simulink model "Dynamic_5R_xd_from_outside"  (R2019a)
settings: Solver=ode3  StartTime=0.0  StopTime=120  FixedStep=0.1  RelTol=1e-3
model workspace (MATLAB code in the model file):
  | fix_step = Simulink.Signal;
  | fix_step.DataType = 'double';
  | fix_step.Dimensions = 1;
  | fix_step.Complexity = 'real';
  | fix_step.SamplingMode = 'Sample based';
  | fix_step.InitialValue = '0.1';
values from neighbouring files (symbols this model uses):
  Kp = 7*eye(2)    [initial_Settings.m]
  Kv = 7*eye(2)    [initial_Settings.m]
  s = 0.0005.*s    [initial_Settings.m]    (also in number2.mat = [129 303 129.214546173 303.585228585 129.437661808 304.16472)
  s1 = [v1;v2]    [initial_Settings.m]
  s2 = [a1;a2]    [initial_Settings.m]
libraries: simulink x1
(part 2 of 2)

== matlab function Dynamic_5R_xd_from_outside/Codes ==
  data: xd input; vd input; ad input; dq input; q input; Kv input; Kp input; x output; t input; xd output; e output; Torque output; wq output; detJ output
function [x,xd,e,Torque,wq,detJ]=  armrobot( xd,vd,ad,dq,q,Kv,Kp,t)



% a1=2.5;
% a2=2.5;
% a3=2.5;
% a4=2.5;
% a5=2.0;


a1=0.25;
a2=0.25;
a3=0.25;
a4=0.25;
a5=0.20;


q2=q(1,1);
q5=q(2,1);

% fprintf('\n  theta2 = %f [rad]  and theta5= %f [rad] \n ' , q2, q5)


A=2*a2*a3*cos(q2)-2*a3*(a5*cos(q5)+a1);
B=2*a2*a3*sin(q2)-2*a3*a5*sin(q5);
C=-1*(-2*a2*(a5*cos(q5)+a1)*cos(q2)+2*a1*a5*cos(q5)-2*a2*sin(q2)*a5*sin(q5)+a1*a1+a2*a2+a3*a3+a5*a5-a4*a4);

t1 = (B+sqrt(A*A+B*B-C*C))/(A+C);

 t2= (B-sqrt(A*A+B*B-C*C))/(A+C);



q3 = 2*atan(t1);
q3 = 2*atan(t2);
q4 = atan2((a2*sin(q2)+a3*sin(q3)-a5*sin(q5)) ,(a2*cos(q2)+a3*cos(q3)-a1-a5*cos(q5)));



wq=[q2;q3;q4;q5];


%%Velocity
w2=dq(1,1);
w5=dq(2,1);


w=inv([-a3*sin(q3) , a4*sin(q4) ; a3*cos(q3) , -a4*cos(q4)])*[a2*w2*sin(q2)-a5*w5*sin(q5) ; -a2*w2*cos(q2)+a5*w5*cos(q5)];

w3=w(1,1);
w4=w(2,1);



%%%%%%%%%%%%%%%%%%%%%%%%%%











%% Acceleration

% alpha2=ddq(1,1);
% alpha5=ddq(2,1);
% 
% t2 = sin(q2);
% t4 = w2 ^ 2;
% t6 = cos(q2);
% t8 = w(1,1) ^ 2;
% t10 = cos(q3);
% t12 = w(2,1) ^ 2;
% t14 = cos(q4);
% t17 = sin(q5);
% t19 = w5 ^ 2;
% t21 = cos(q5);
% A1 = a2 * alpha2 * t2 + a2 * t4 * t6 + a3 * t8 * t10 - a4 * t12 * t14 - a5 * alpha5 * t17 - a5 * t19 * t21;
% 
% 
% t2 = cos(q2);
% t4 = w2 ^ 2;
% t6 = sin(q2);
% t8 = w(1,1) ^ 2;
% t10 = sin(q3);
% t12 = w(2,1) ^ 2;
% t14 = sin(q4);
% t17 = cos(q5);
% t19 = w5 ^ 2;
% t21 = sin(q5);
% A2 = -a2 * alpha2 * t2 + a2 * t4 * t6 + a3 * t8 * t10 - a4 * t12 * t14 + a5 * alpha5 * t17 - a5 * t19 * t21;
% 
% 
% 
% % This gives us alpha3 and alpha4
% alpha= inv([-a3*sin(q3) , a4*sin(q4) ; a3*cos(q3) , -a4*cos(q4)])*[A1;A2]
% 
% 


%% Jacobian Matrices
%Link2
% --------------------------------------------------------------
Jplink2=[-a2*0.5*sin(q2),0;a2*cos(q2)*0.5 , 0 ; 0, 0]
Jolink2=[0,0;0,0;1,0];
% --------------------------------------------------------------

%Link3
% --------------------------------------------------------------


%%Derivative theta3 wrt theta2
t1 = a3 * a2;
t2 = cos(q2);
t3 = t2 * t1;
t4 = 0.2e1 * t3;
t5 = cos(q5);
t7 = t5 * a5 + a1;
t8 = t7 * a3;
t9 = t3 - t8;
t11 = sin(q2);
t12 = t11 * t1;
t13 = sin(q5);
t15 = a5 * a3 * t13;
t16 = t12 - t15;
t18 = t7 * a2;
t20 = 0.2e1 * t2 * t18;
t23 = 0.2e1 * a5 * a1 * t5;
t25 = a2 * a5;
t27 = 0.2e1 * t25 * t13 * t11;
t28 = a1 ^ 2;
t29 = a2 ^ 2;
t30 = a3 ^ 2;
t31 = a5 ^ 2;
t32 = a4 ^ 2;
t33 = t20 - t23 + t27 - t28 - t29 - t30 - t31 + t32;
t34 = t33 ^ 2;
t36 = sqrt(0.4e1 * t16 ^ 2 + 0.4e1 * t9 ^ 2 - t34);
t46 = t11 * t18;
t48 = t25 * t13 * t2;
t57 = t4 - 0.2e1 * t8 + t20 - t23 + t27 - t28 - t29 - t30 - t31 + t32;
t62 = 0.2e1 * t12 - 0.2e1 * t15 - t36;
t63 = t57 ^ 2;
t64 = 0.1e1 / t63;
t69 = t62 ^ 2;
derivative_q3_wrt_q2= 0.2e1 / (t64 * t69 + 0.1e1) * (0.1e1 / t57 * (t4 - (-0.8e1 * t11 * a3 * a2 * t9 + 0.8e1 * t2 * a3 * a2 * t16 - 0.4e1 * (-t46 + t48) * t33) / t36 / 0.2e1) - 0.2e1 * (-t12 - t46 + t48) * t64 * t62);



%%Derivative theta3 wrt theta5


t1 = cos(q5);
t5 = a3 * a2;
t6 = cos(q2);
t7 = t6 * t5;
t9 = t1 * a5 + a1;
t10 = t9 * a3;
t11 = t7 - t10;
t13 = sin(q2);
t14 = t13 * t5;
t15 = sin(q5);
t17 = a5 * a3 * t15;
t18 = t14 - t17;
t22 = 0.2e1 * t6 * t9 * a2;
t25 = 0.2e1 * a5 * a1 * t1;
t27 = a2 * a5;
t29 = 0.2e1 * t27 * t15 * t13;
t30 = a1 ^ 2;
t31 = a2 ^ 2;
t32 = a3 ^ 2;
t33 = a5 ^ 2;
t34 = a4 ^ 2;
t35 = t22 - t25 + t29 - t30 - t31 - t32 - t33 + t34;
t36 = t35 ^ 2;
t38 = sqrt(0.4e1 * t11 ^ 2 + 0.4e1 * t18 ^ 2 - t36);
t41 = a3 * a5;
t48 = t27 * t15 * t6;
t50 = a5 * a1 * t15;
t52 = t27 * t1 * t13;
t62 = 0.2e1 * t7 - 0.2e1 * t10 + t22 - t25 + t29 - t30 - t31 - t32 - t33 + t34;
t67 = 0.2e1 * t14 - 0.2e1 * t17 - t38;
t68 = t62 ^ 2;
t69 = 0.1e1 / t68;
t74 = t67 ^ 2;
derivative_q3_wrt_q5 = 0.2e1 / (t69 * t74 + 0.1e1) * (0.1e1 / t62 * (-0.2e1 * a5 * a3 * t1 - (0.8e1 * t41 * t15 * t11 - 0.8e1 * t41 * t1 * t18 - 0.4e1 * (-t48 + t50 + t52) * t35) / t38 / 0.2e1) - 0.2e1 * (t17 - t48 + t50 + t52) * t69 * t67);






Jplink3=[-a2*sin(q2)-a3*0.5*sin(q3)*derivative_q3_wrt_q2 , -a3*0.5*sin(q3)*derivative_q3_wrt_q5 ;
          a2*cos(q2)+a3*0.5*cos(q3)*derivative_q3_wrt_q2 , a3*0.5*cos(q3)*derivative_q3_wrt_q5;
           0     , 0];

Jolink3=[0,0;0,0;derivative_q3_wrt_q2,derivative_q3_wrt_q5];
% --------------------------------------------------------------


% link4
% --------------------------------------------------------------
%%Derivative theta4 wrt theta2
t1 = cos(q2);
t2 = a2 * t1;
t3 = a3 * a2;
t4 = t1 * t3;
t5 = 0.2e1 * t4;
t6 = cos(q5);
t7 = t6 * a5;
t8 = t7 + a1;
t9 = t8 * a3;
t10 = t4 - t9;
t12 = sin(q2);
t13 = t12 * t3;
t14 = sin(q5);
t16 = a5 * a3 * t14;
t17 = t13 - t16;
t19 = t8 * a2;
t21 = 0.2e1 * t1 * t19;
t24 = 0.2e1 * a5 * a1 * t6;
t26 = a2 * a5;
t28 = 0.2e1 * t26 * t14 * t12;
t29 = a1 ^ 2;
t30 = a2 ^ 2;
t31 = a3 ^ 2;
t32 = a5 ^ 2;
t33 = a4 ^ 2;
t34 = t21 - t24 + t28 - t29 - t30 - t31 - t32 + t33;
t35 = t34 ^ 2;
t37 = sqrt(0.4e1 * t10 ^ 2 + 0.4e1 * t17 ^ 2 - t35);
t47 = t12 * t19;
t49 = t26 * t14 * t1;
t58 = t5 - 0.2e1 * t9 + t21 - t24 + t28 - t29 - t30 - t31 - t32 + t33;
t59 = 0.1e1 / t58;
t63 = 0.2e1 * t13 - 0.2e1 * t16 - t37;
t64 = t58 ^ 2;
t65 = 0.1e1 / t64;
t70 = (t59 * (t5 - (-0.8e1 * t12 * a3 * a2 * t10 + 0.8e1 * t1 * a3 * a2 * t17 - 0.4e1 * (-t47 + t49) * t34) / t37 / 0.2e1) - 0.2e1 * (-t13 - t47 + t49) * t65 * t63) * a3;
t71 = t63 ^ 2;
t74 = 0.1e1 / (t65 * t71 + 0.1e1);
t76 = atan(t59 * t63);
t77 = 0.2e1 * t76;
t78 = cos(t77);
t84 = t78 * a3 - a1 + t2 - t7;
t87 = t12 * a2;
t88 = sin(t77);
t91 = t88 * a3 - t14 * a5 + t87;
t92 = t91 ^ 2;
t93 = t84 ^ 2;
t94 = 0.1e1 / t93;
t97 = 0.1e1 / (t94 * t92 + 0.1e1);
derivative_q4_wrt_q2 = t97 / t84 * (0.2e1 * t78 * t74 * t70 + t2) - t97 * t94 * t91 * (-0.2e1 * t88 * t74 * t70 - t87);





%%Derivative theta4 wrt theta5


t1 = cos(q5);
t5 = a3 * a2;
t6 = cos(q2);
t7 = t6 * t5;
t8 = t1 * a5;
t9 = t8 + a1;
t10 = t9 * a3;
t11 = t7 - t10;
t13 = sin(q2);
t14 = t13 * t5;
t15 = sin(q5);
t17 = a5 * a3 * t15;
t18 = t14 - t17;
t22 = 0.2e1 * t6 * t9 * a2;
t25 = 0.2e1 * a5 * a1 * t1;
t27 = a2 * a5;
t29 = 0.2e1 * t27 * t15 * t13;
t30 = a1 ^ 2;
t31 = a2 ^ 2;
t32 = a3 ^ 2;
t33 = a5 ^ 2;
t34 = a4 ^ 2;
t35 = t22 - t25 + t29 - t30 - t31 - t32 - t33 + t34;
t36 = t35 ^ 2;
t38 = sqrt(0.4e1 * t11 ^ 2 + 0.4e1 * t18 ^ 2 - t36);
t41 = a3 * a5;
t48 = t27 * t15 * t6;
t50 = a5 * a1 * t15;
t52 = t27 * t1 * t13;
t62 = 0.2e1 * t7 - 0.2e1 * t10 + t22 - t25 + t29 - t30 - t31 - t32 - t33 + t34;
t63 = 0.1e1 / t62;
t67 = 0.2e1 * t14 - 0.2e1 * t17 - t38;
t68 = t62 ^ 2;
t69 = 0.1e1 / t68;
t74 = ((-0.2e1 * a5 * a3 * t1 - (0.8e1 * t41 * t15 * t11 - 0.8e1 * t41 * t1 * t18 - 0.4e1 * (-t48 + t50 + t52) * t35) / t38 / 0.2e1) * t63 - 0.2e1 * (t17 - t48 + t50 + t52) * t69 * t67) * a3;
t75 = t67 ^ 2;
t78 = 0.1e1 / (t69 * t75 + 0.1e1);
t80 = atan(t63 * t67);
t81 = 0.2e1 * t80;
t82 = cos(t81);
t89 = a2 * t6 + t82 * a3 - a1 - t8;
t93 = sin(t81);
t95 = t15 * a5;
t96 = t13 * a2 + t93 * a3 - t95;
t97 = t96 ^ 2;
t98 = t89 ^ 2;
t99 = 0.1e1 / t98;
t102 = 0.1e1 / (t99 * t97 + 0.1e1);
derivative_q4_wrt_q5= 0.1e1 / t89 * (0.2e1 * t82 * t78 * t74 - t8) * t102 - t102 * t99 * t96 * (-0.2e1 * t93 * t78 * t74 + t95);

Jplink4=[-a4*0.5*sin(q4)*derivative_q4_wrt_q2 , -a5*sin(q5)-a4*0.5*sin(q4)*derivative_q4_wrt_q5 ;
         a4*0.5*cos(q4)*derivative_q4_wrt_q2 , a5*cos(q5)+a4*0.5*cos(q4)*derivative_q4_wrt_q5 ; 0,0];


     
Jolink4=[0,0 ; 0,0 ; derivative_q4_wrt_q2 ,derivative_q4_wrt_q5];     
     
% link5   
Jplink5=[0,-a5*0.5*sin(q5) ; 0 ,a5*0.5*cos(q5) ; 0 ,0];
Jolink5=[0,0;0,0;0,1];










%%Second Derivatives


% Derivative of function q3 with respect to q2 q2


t1 = a2 * a3;
t2 = sin(q2);
t3 = t2 * t1;
t4 = 0.2e1 * t3;
t5 = cos(q2);
t6 = t5 * t1;
t7 = cos(q5);
t9 = t7 * a5 + a1;
t10 = t9 * a3;
t11 = t6 - t10;
t12 = 0.2e1 * a2 * t11;
t13 = t2 * a3;
t16 = sin(q5);
t18 = a5 * a3 * t16;
t19 = t3 - t18;
t20 = 0.2e1 * a2 * t19;
t21 = t5 * a3;
t24 = t9 * a2;
t25 = t5 * t24;
t26 = 0.2e1 * t25;
t29 = 0.2e1 * a5 * a1 * t7;
t31 = a2 * a5;
t32 = t31 * t16 * t2;
t33 = 0.2e1 * t32;
t34 = a1 ^ 2;
t35 = a2 ^ 2;
t36 = a3 ^ 2;
t37 = a5 ^ 2;
t38 = a4 ^ 2;
t39 = t26 - t29 + t33 - t34 - t35 - t36 - t37 + t38;
t40 = t2 * t24;
t42 = t31 * t16 * t5;
t43 = -t40 + t42;
t46 = -0.4e1 * t13 * t12 + 0.4e1 * t21 * t20 - 0.4e1 * t43 * t39;
t47 = t46 ^ 2;
t50 = t39 ^ 2;
t51 = 0.4e1 * t11 ^ 2 + 0.4e1 * t19 ^ 2 - t50;
t52 = sqrt(t51);
t57 = t2 ^ 2;
t63 = t5 ^ 2;
t75 = 0.1e1 / t52;
t79 = 0.2e1 * t6;
t81 = t79 - 0.2e1 * t10 + t26 - t29 + t33 - t34 - t35 - t36 - t37 + t38;
t82 = 0.1e1 / t81;
t86 = t79 - t75 * t46 / 0.2e1;
t87 = -t3 - t40 + t42;
t89 = t81 ^ 2;
t90 = 0.1e1 / t89;
t94 = t4 - 0.2e1 * t18 - t52;
t98 = 0.1e1 / t89 / t81;
t105 = t94 ^ 2;
t107 = t90 * t105 + 0.1e1;
t120 = t107 ^ 2;
derivative_q3_wrt_q2_q2 = 0.2e1 / t107 * (t82 * (-t4 + 0.1e1 / t52 / t51 * t47 / 0.4e1 - t75 * (0.8e1 * t36 * t35 * t57 - 0.4e1 * t21 * t12 + 0.8e1 * t36 * t35 * t63 - 0.4e1 * t13 * t20 - 0.8e1 * t43 ^ 2 - 0.4e1 * (-t25 - t32) * t39) / 0.2e1) - 0.4e1 * t90 * t87 * t86 + 0.8e1 * t98 * t87 ^ 2 * t94 - 0.2e1 * t90 * (-t6 - t25 - t32) * t94) - 0.4e1 / t120 * (-0.2e1 * t98 * t87 * t105 + t90 * t86 * t94) * (-0.2e1 * t90 * t87 * t94 + t82 * t86);





% derivative q3 with respecto q2 q5



t1 = a3 * a2;
t2 = cos(q2);
t3 = t2 * t1;
t4 = cos(q5);
t6 = t4 * a5 + a1;
t7 = t6 * a3;
t8 = t3 - t7;
t10 = sin(q2);
t14 = t10 * t1;
t15 = sin(q5);
t17 = a5 * a3 * t15;
t18 = t14 - t17;
t23 = t6 * a2;
t25 = 0.2e1 * t2 * t23;
t28 = 0.2e1 * a5 * a1 * t4;
t29 = t15 * t10;
t30 = a2 * a5;
t31 = t30 * t29;
t32 = 0.2e1 * t31;
t33 = a1 ^ 2;
t34 = a2 ^ 2;
t35 = a3 ^ 2;
t36 = a5 ^ 2;
t37 = a4 ^ 2;
t38 = t25 - t28 + t32 - t33 - t34 - t35 - t36 + t37;
t39 = t10 * t23;
t41 = t30 * t15 * t2;
t42 = -t39 + t41;
t45 = -0.8e1 * t10 * a3 * a2 * t8 + 0.8e1 * t2 * a3 * a2 * t18 - 0.4e1 * t42 * t38;
t47 = a3 * a5;
t54 = a5 * a1 * t15;
t56 = t30 * t4 * t10;
t57 = -t41 + t54 + t56;
t60 = 0.8e1 * t47 * t15 * t8 - 0.8e1 * t47 * t4 * t18 - 0.4e1 * t57 * t38;
t64 = t38 ^ 2;
t65 = 0.4e1 * t18 ^ 2 + 0.4e1 * t8 ^ 2 - t64;
t66 = sqrt(t65);
t72 = a5 * t35 * a2;
t75 = t4 * t2;
t81 = t30 * t75 + t31;
t85 = 0.1e1 / t66;
t89 = 0.2e1 * t3;
t91 = t89 - 0.2e1 * t7 + t25 - t28 + t32 - t33 - t34 - t35 - t36 + t37;
t92 = 0.1e1 / t91;
t96 = t89 - t85 * t45 / 0.2e1;
t97 = t17 - t41 + t54 + t56;
t99 = t91 ^ 2;
t100 = 0.1e1 / t99;
t107 = -0.2e1 * a5 * a3 * t4 - t85 * t60 / 0.2e1;
t108 = -t14 - t39 + t41;
t113 = 0.2e1 * t14 - 0.2e1 * t17 - t66;
t114 = 0.2e1 * t108 * t113;
t116 = 0.1e1 / t99 / t91;
t123 = t113 ^ 2;
t125 = t100 * t123 + 0.1e1;
t137 = t125 ^ 2;
derivative_q3_wrt_q2_q5 = 0.2e1 / t125 * (t92 * (0.1e1 / t66 / t65 * t60 * t45 / 0.4e1 - t85 * (-0.8e1 * t72 * t29 - 0.4e1 * t81 * t38 - 0.8e1 * t42 * t57 - 0.8e1 * t72 * t75) / 0.2e1) - 0.2e1 * t100 * t97 * t96 - 0.2e1 * t100 * t108 * t107 + 0.4e1 * t116 * t97 * t114 - 0.2e1 * t100 * t81 * t113) - 0.4e1 / t137 * (t100 * t107 * t113 - 0.2e1 * t116 * t97 * t123) * (-t100 * t114 + t92 * t96);


%derivative q3 with respecto q5 q5

t1 = sin(q5);
t3 = a5 * a3 * t1;
t4 = 0.2e1 * t3;
t5 = a2 * a3;
t6 = cos(q2);
t7 = t6 * t5;
t8 = cos(q5);
t10 = t8 * a5 + a1;
t11 = t10 * a3;
t12 = t7 - t11;
t14 = a3 * a5;
t17 = sin(q2);
t18 = t17 * t5;
t19 = t18 - t3;
t25 = 0.2e1 * t6 * t10 * a2;
t27 = a5 * a1 * t8;
t28 = 0.2e1 * t27;
t30 = a2 * a5;
t31 = t30 * t1 * t17;
t32 = 0.2e1 * t31;
t33 = a1 ^ 2;
t34 = a2 ^ 2;
t35 = a3 ^ 2;
t36 = a5 ^ 2;
t37 = a4 ^ 2;
t38 = t25 - t28 + t32 - t33 - t34 - t35 - t36 + t37;
t40 = t30 * t1 * t6;
t42 = a5 * a1 * t1;
t44 = t30 * t8 * t17;
t45 = -t40 + t42 + t44;
t48 = 0.8e1 * t14 * t1 * t12 - 0.8e1 * t14 * t8 * t19 - 0.4e1 * t45 * t38;
t49 = t48 ^ 2;
t52 = t38 ^ 2;
t53 = 0.4e1 * t12 ^ 2 + 0.4e1 * t19 ^ 2 - t52;
t54 = sqrt(t53);
t59 = t1 ^ 2;
t66 = t8 ^ 2;
t76 = t30 * t8 * t6;
t81 = 0.1e1 / t54;
t87 = 0.2e1 * t7 - 0.2e1 * t11 + t25 - t28 + t32 - t33 - t34 - t35 - t36 + t37;
t88 = 0.1e1 / t87;
t91 = a5 * a3 * t8;
t95 = -0.2e1 * t91 - t81 * t48 / 0.2e1;
t96 = t3 - t40 + t42 + t44;
t98 = t87 ^ 2;
t99 = 0.1e1 / t98;
t103 = 0.2e1 * t18 - t4 - t54;
t107 = 0.1e1 / t98 / t87;
t114 = t103 ^ 2;
t116 = t99 * t114 + 0.1e1;
t129 = t116 ^ 2;
derivative_q3_wrt_q5_q5 = 0.2e1 / t116 * (t88 * (t4 + 0.1e1 / t54 / t53 * t49 / 0.4e1 - t81 * (0.8e1 * t36 * t35 * t59 + 0.8e1 * t14 * t8 * t12 + 0.8e1 * t36 * t35 * t66 + 0.8e1 * t14 * t1 * t19 - 0.8e1 * t45 ^ 2 - 0.4e1 * (-t76 + t27 - t31) * t38) / 0.2e1) - 0.4e1 * t99 * t96 * t95 + 0.8e1 * t107 * t96 ^ 2 * t103 - 0.2e1 * t99 * (t91 - t76 + t27 - t31) * t103) - 0.4e1 / t129 * (t99 * t95 * t103 - 0.2e1 * t107 * t96 * t114) * (-0.2e1 * t99 * t96 * t103 + t88 * t95);

%%%%



%-------------------------------------------------
% derivative theta4 with respect to theta2 theta2

t1 = sin(q2);
t2 = t1 * a2;
t3 = a3 * a2;
t4 = t1 * t3;
t5 = 0.2e1 * t4;
t6 = cos(q2);
t7 = t6 * t3;
t8 = cos(q5);
t9 = t8 * a5;
t10 = t9 + a1;
t11 = t10 * a3;
t12 = t7 - t11;
t13 = 0.2e1 * a2 * t12;
t14 = t1 * a3;
t17 = sin(q5);
t19 = a5 * a3 * t17;
t20 = t4 - t19;
t21 = 0.2e1 * a2 * t20;
t22 = t6 * a3;
t25 = t10 * a2;
t26 = t6 * t25;
t27 = 0.2e1 * t26;
t30 = 0.2e1 * a5 * a1 * t8;
t32 = a2 * a5;
t33 = t32 * t17 * t1;
t34 = 0.2e1 * t33;
t35 = a1 ^ 2;
t36 = a2 ^ 2;
t37 = a3 ^ 2;
t38 = a5 ^ 2;
t39 = a4 ^ 2;
t40 = t27 - t30 + t34 - t35 - t36 - t37 - t38 + t39;
t41 = t1 * t25;
t43 = t32 * t17 * t6;
t44 = -t41 + t43;
t47 = -0.4e1 * t14 * t13 + 0.4e1 * t22 * t21 - 0.4e1 * t44 * t40;
t48 = t47 ^ 2;
t51 = t40 ^ 2;
t52 = 0.4e1 * t12 ^ 2 + 0.4e1 * t20 ^ 2 - t51;
t53 = sqrt(t52);
t58 = t1 ^ 2;
t64 = t6 ^ 2;
t76 = 0.1e1 / t53;
t80 = 0.2e1 * t7;
t82 = t80 - 0.2e1 * t11 + t27 - t30 + t34 - t35 - t36 - t37 - t38 + t39;
t83 = 0.1e1 / t82;
t87 = t80 - t76 * t47 / 0.2e1;
t88 = -t4 - t41 + t43;
t90 = t82 ^ 2;
t91 = 0.1e1 / t90;
t95 = t5 - 0.2e1 * t19 - t53;
t99 = 0.1e1 / t90 / t82;
t106 = (t83 * (-t5 + 0.1e1 / t53 / t52 * t48 / 0.4e1 - t76 * (0.8e1 * t37 * t36 * t58 - 0.4e1 * t22 * t13 + 0.8e1 * t37 * t36 * t64 - 0.4e1 * t14 * t21 - 0.8e1 * t44 ^ 2 - 0.4e1 * (-t26 - t33) * t40) / 0.2e1) - 0.4e1 * t91 * t88 * t87 + 0.8e1 * t99 * t88 ^ 2 * t95 - 0.2e1 * t91 * (-t7 - t26 - t33) * t95) * a3;
t108 = atan(t83 * t95);
t109 = 0.2e1 * t108;
t110 = cos(t109);
t111 = t95 ^ 2;
t113 = t91 * t111 + 0.1e1;
t114 = 0.1e1 / t113;
t115 = t114 * t110;
t121 = -0.2e1 * t91 * t88 * t95 + t83 * t87;
t122 = t121 * a3;
t127 = -0.2e1 * t99 * t88 * t111 + t91 * t87 * t95;
t129 = t113 ^ 2;
t130 = 0.1e1 / t129;
t134 = t121 ^ 2;
t135 = t134 * a3;
t136 = sin(t109);
t141 = t6 * a2;
t143 = t110 * a3 - a1 + t141 - t9;
t144 = 0.1e1 / t143;
t148 = t136 * a3 - t17 * a5 + t2;
t149 = t148 ^ 2;
t150 = t143 ^ 2;
t151 = 0.1e1 / t150;
t153 = t151 * t149 + 0.1e1;
t154 = 0.1e1 / t153;
t158 = 0.2e1 * t115 * t122 + t141;
t159 = t114 * t136;
t162 = -0.2e1 * t159 * t122 - t2;
t164 = t154 * t151;
t171 = 0.1e1 / t150 / t143;
t173 = t151 * t158 * t148 - t171 * t162 * t149;
t175 = t153 ^ 2;
t176 = 0.1e1 / t175;
t191 = t162 ^ 2;
derivative_q4_wrt_q2_q2 = t154 * t144 * (-0.4e1 * t130 * t127 * t110 * t122 - 0.4e1 * t130 * t136 * t135 + 0.2e1 * t115 * t106 - t2) - 0.2e1 * t164 * t162 * t158 - 0.2e1 * t176 * t144 * t173 * t158 - t164 * t148 * (0.4e1 * t130 * t127 * t136 * t122 - 0.4e1 * t130 * t110 * t135 - 0.2e1 * t159 * t106 - t141) + 0.2e1 * t154 * t171 * t148 * t191 + 0.2e1 * t176 * t151 * t173 * t148 * t162;

%-------------------------------------------------------------
% derivative theta4 with respect to theta2 theta5




t1 = a3 * a2;
t2 = cos(q2);
t3 = t2 * t1;
t4 = cos(q5);
t5 = t4 * a5;
t6 = t5 + a1;
t7 = t6 * a3;
t8 = t3 - t7;
t10 = sin(q2);
t14 = t10 * t1;
t15 = sin(q5);
t17 = a5 * a3 * t15;
t18 = t14 - t17;
t23 = t6 * a2;
t25 = 0.2e1 * t2 * t23;
t28 = 0.2e1 * a5 * a1 * t4;
t29 = t15 * t10;
t30 = a2 * a5;
t31 = t30 * t29;
t32 = 0.2e1 * t31;
t33 = a1 ^ 2;
t34 = a2 ^ 2;
t35 = a3 ^ 2;
t36 = a5 ^ 2;
t37 = a4 ^ 2;
t38 = t25 - t28 + t32 - t33 - t34 - t35 - t36 + t37;
t39 = t10 * t23;
t41 = t30 * t15 * t2;
t42 = -t39 + t41;
t45 = -0.8e1 * t10 * a3 * a2 * t8 + 0.8e1 * t2 * a3 * a2 * t18 - 0.4e1 * t42 * t38;
t47 = a3 * a5;
t54 = a5 * a1 * t15;
t56 = t30 * t4 * t10;
t57 = -t41 + t54 + t56;
t60 = 0.8e1 * t47 * t15 * t8 - 0.8e1 * t47 * t4 * t18 - 0.4e1 * t57 * t38;
t64 = t38 ^ 2;
t65 = 0.4e1 * t18 ^ 2 + 0.4e1 * t8 ^ 2 - t64;
t66 = sqrt(t65);
t72 = a5 * t35 * a2;
t75 = t4 * t2;
t81 = t30 * t75 + t31;
t85 = 0.1e1 / t66;
t89 = 0.2e1 * t3;
t91 = t89 - 0.2e1 * t7 + t25 - t28 + t32 - t33 - t34 - t35 - t36 + t37;
t92 = 0.1e1 / t91;
t96 = t89 - t85 * t45 / 0.2e1;
t97 = t17 - t41 + t54 + t56;
t99 = t91 ^ 2;
t100 = 0.1e1 / t99;
t107 = -0.2e1 * a5 * a3 * t4 - t85 * t60 / 0.2e1;
t108 = -t14 - t39 + t41;
t113 = 0.2e1 * t14 - 0.2e1 * t17 - t66;
t114 = 0.2e1 * t108 * t113;
t116 = 0.1e1 / t99 / t91;
t123 = (t92 * (0.1e1 / t66 / t65 * t60 * t45 / 0.4e1 - t85 * (-0.8e1 * t72 * t29 - 0.4e1 * t81 * t38 - 0.8e1 * t42 * t57 - 0.8e1 * t72 * t75) / 0.2e1) - 0.2e1 * t100 * t97 * t96 - 0.2e1 * t100 * t108 * t107 + 0.4e1 * t116 * t97 * t114 - 0.2e1 * t100 * t81 * t113) * a3;
t125 = atan(t92 * t113);
t126 = 0.2e1 * t125;
t127 = cos(t126);
t128 = t113 ^ 2;
t130 = t100 * t128 + 0.1e1;
t131 = 0.1e1 / t130;
t132 = t131 * t127;
t138 = (-t100 * t114 + t92 * t96) * a3;
t143 = t100 * t107 * t113 - 0.2e1 * t116 * t97 * t128;
t145 = t130 ^ 2;
t146 = 0.1e1 / t145;
t153 = -0.2e1 * t100 * t97 * t113 + t92 * t107;
t154 = sin(t126);
t160 = t2 * a2;
t162 = t127 * a3 - a1 + t160 - t5;
t163 = 0.1e1 / t162;
t165 = t10 * a2;
t167 = t15 * a5;
t168 = t154 * a3 + t165 - t167;
t169 = t168 ^ 2;
t170 = t162 ^ 2;
t171 = 0.1e1 / t170;
t173 = t171 * t169 + 0.1e1;
t174 = 0.1e1 / t173;
t178 = 0.2e1 * t132 * t138 + t160;
t179 = t153 * a3;
t180 = t131 * t154;
t183 = -0.2e1 * t180 * t179 + t167;
t185 = t174 * t171;
t189 = 0.2e1 * t132 * t179 - t5;
t194 = 0.1e1 / t170 / t162;
t196 = t171 * t189 * t168 - t194 * t183 * t169;
t198 = t173 ^ 2;
t199 = 0.1e1 / t198;
t217 = -0.2e1 * t180 * t138 - t165;
t220 = t168 * t217;
derivative_q4_wrt_q2_q5 = t174 * t163 * (-0.4e1 * t146 * t143 * t127 * t138 - 0.4e1 * t146 * t154 * t153 * t138 + 0.2e1 * t132 * t123) - t185 * t183 * t178 - 0.2e1 * t199 * t163 * t196 * t178 - t185 * t168 * (-0.4e1 * t146 * t127 * t153 * t138 + 0.4e1 * t146 * t143 * t154 * t138 - 0.2e1 * t180 * t123) - t185 * t189 * t217 + 0.2e1 * t174 * t194 * t183 * t220 + 0.2e1 * t199 * t171 * t196 * t220;

%derivative q4 with respect to q5 q5
%---------------------------------------------------------

t1 = sin(q5);
t3 = a5 * a3 * t1;
t4 = 0.2e1 * t3;
t5 = a3 * a2;
t6 = cos(q2);
t7 = t6 * t5;
t8 = cos(q5);
t9 = t8 * a5;
t10 = t9 + a1;
t11 = t10 * a3;
t12 = t7 - t11;
t14 = a3 * a5;
t17 = sin(q2);
t18 = t17 * t5;
t19 = t18 - t3;
t25 = 0.2e1 * t6 * t10 * a2;
t27 = a5 * a1 * t8;
t28 = 0.2e1 * t27;
t30 = a2 * a5;
t31 = t30 * t1 * t17;
t32 = 0.2e1 * t31;
t33 = a1 ^ 2;
t34 = a2 ^ 2;
t35 = a3 ^ 2;
t36 = a5 ^ 2;
t37 = a4 ^ 2;
t38 = t25 - t28 + t32 - t33 - t34 - t35 - t36 + t37;
t40 = t30 * t1 * t6;
t42 = a5 * a1 * t1;
t44 = t30 * t8 * t17;
t45 = -t40 + t42 + t44;
t48 = 0.8e1 * t14 * t1 * t12 - 0.8e1 * t14 * t8 * t19 - 0.4e1 * t45 * t38;
t49 = t48 ^ 2;
t52 = t38 ^ 2;
t53 = 0.4e1 * t12 ^ 2 + 0.4e1 * t19 ^ 2 - t52;
t54 = sqrt(t53);
t59 = t1 ^ 2;
t66 = t8 ^ 2;
t76 = t30 * t8 * t6;
t81 = 0.1e1 / t54;
t87 = 0.2e1 * t7 - 0.2e1 * t11 + t25 - t28 + t32 - t33 - t34 - t35 - t36 + t37;
t88 = 0.1e1 / t87;
t91 = a5 * a3 * t8;
t95 = -0.2e1 * t91 - t81 * t48 / 0.2e1;
t96 = t3 - t40 + t42 + t44;
t98 = t87 ^ 2;
t99 = 0.1e1 / t98;
t103 = 0.2e1 * t18 - t4 - t54;
t107 = 0.1e1 / t98 / t87;
t114 = (t88 * (t4 + 0.1e1 / t54 / t53 * t49 / 0.4e1 - t81 * (0.8e1 * t36 * t35 * t59 + 0.8e1 * t14 * t8 * t12 + 0.8e1 * t36 * t35 * t66 + 0.8e1 * t14 * t1 * t19 - 0.8e1 * t45 ^ 2 - 0.4e1 * (-t76 + t27 - t31) * t38) / 0.2e1) - 0.4e1 * t99 * t96 * t95 + 0.8e1 * t107 * t96 ^ 2 * t103 - 0.2e1 * t99 * (t91 - t76 + t27 - t31) * t103) * a3;
t116 = atan(t88 * t103);
t117 = 0.2e1 * t116;
t118 = cos(t117);
t119 = t103 ^ 2;
t121 = t99 * t119 + 0.1e1;
t122 = 0.1e1 / t121;
t123 = t122 * t118;
t129 = -0.2e1 * t99 * t96 * t103 + t88 * t95;
t130 = t129 * a3;
t135 = t99 * t95 * t103 - 0.2e1 * t107 * t96 * t119;
t137 = t121 ^ 2;
t138 = 0.1e1 / t137;
t142 = t129 ^ 2;
t143 = t142 * a3;
t144 = sin(t117);
t148 = t1 * a5;
t152 = t6 * a2 + t118 * a3 - a1 - t9;
t153 = 0.1e1 / t152;
t157 = t17 * a2 + t144 * a3 - t148;
t158 = t157 ^ 2;
t159 = t152 ^ 2;
t160 = 0.1e1 / t159;
t162 = t160 * t158 + 0.1e1;
t163 = 0.1e1 / t162;
t167 = 0.2e1 * t123 * t130 - t9;
t168 = t122 * t144;
t171 = -0.2e1 * t168 * t130 + t148;
t173 = t163 * t160;
t180 = 0.1e1 / t159 / t152;
t182 = t160 * t167 * t157 - t180 * t171 * t158;
t184 = t162 ^ 2;
t185 = 0.1e1 / t184;
t200 = t171 ^ 2;
derivative_q4_wrt_q5_q5= t163 * t153 * (-0.4e1 * t138 * t135 * t118 * t130 - 0.4e1 * t138 * t144 * t143 + 0.2e1 * t123 * t114 + t148) - 0.2e1 * t173 * t171 * t167 - 0.2e1 * t185 * t153 * t182 * t167 - t173 * t157 * (0.4e1 * t138 * t135 * t144 * t130 - 0.4e1 * t138 * t118 * t143 - 0.2e1 * t168 * t114 + t9) + 0.2e1 * t163 * t180 * t157 * t200 + 0.2e1 * t185 * t160 * t182 * t157 * t171;


%% Inertia Tensors for all links

Inertia_link2=2*eye(3);
Inertia_link3=2*eye(3);
Inertia_link4=2*eye(3);
Inertia_link5=1.3*eye(3);



%%Mass Matrix
m2=0.85;
m3=0.85;
m4=0.85;
m5=0.75;


% Rotation Matrix
% [cos(q),-sin(q),0 ;sin(q),cos(q),0 ; 0,0,1]

% M=m2*transpose(Jplink2)*Jplink2+transpose(Jolink2)*[cos(q2),-sin(q2),0 ;sin(q2),cos(q2),0 ; 0,0,1]*Inertia_link2*transpose([cos(q2),-sin(q2),0 ;sin(q2),cos(q2),0 ; 0,0,1])*Jolink2 ...
%   +m3*transpose(Jplink3)*Jplink3+transpose(Jolink3)*[cos(q3),-sin(q3),0 ;sin(q3),cos(q3),0 ; 0,0,1]*Inertia_link3*transpose([cos(q3),-sin(q3),0 ;sin(q3),cos(q3),0 ; 0,0,1])*Jolink3 ...
%   +m4*transpose(Jplink4)*Jplink4+transpose(Jolink4)*[cos(q4),-sin(q4),0 ;sin(q4),cos(q4),0 ; 0,0,1]*Inertia_link4*transpose([cos(q4),-sin(q4),0 ;sin(q4),cos(q4),0 ; 0,0,1])*Jolink4 ...
%   +m5*transpose(Jplink5)*Jplink5+transpose(Jolink5)*[cos(q5),-sin(q5),0 ;sin(q5),cos(q5),0 ; 0,0,1]*Inertia_link5*transpose([cos(q5),-sin(q5),0 ;sin(q5),cos(q5),0 ; 0,0,1])*Jolink5
% 




Izz2=Inertia_link2(3,3);
Izz3=Inertia_link3(3,3);
Izz4=Inertia_link4(3,3);
Izz5=Inertia_link5(3,3);
%%Mass Matrix

% Summation index 2
t1 = sin(q2);
t2 = cos(q2);
Mass_matrix_2 = [m2 * a2 ^ 2 * (t1 ^ 2 + t2 ^ 2) / 0.4e1 + Izz2 0; 0 0;];


% Summation index 3
t1 = q3;
t2 = sin(t1);
t3 = a3 * derivative_q3_wrt_q2/ 0.2e1;
t4 = -a2 * sin(q2) - t3 * t2;
t1 = cos(t1);
t3 = a2 * cos(q2) + t3 * t1;
t5 = -m3 * a3 * derivative_q3_wrt_q5 * (-t3 * t1 + t2 * t4) / 0.2e1 + derivative_q3_wrt_q2 * Izz3 * derivative_q3_wrt_q5;
t6 = derivative_q3_wrt_q5 ^ 2;
Mass_matrix_3 = [derivative_q3_wrt_q2 ^ 2 * Izz3 + (t3 ^ 2 + t4 ^ 2) * m4 t5; t5 t6 * Izz3 + a3 ^ 2 * m4 * t6 * (t1 ^ 2 + t2 ^ 2) / 0.4e1;];

% Summation index 4

t1 = q4;
t2 = sin(t1);
t1 = cos(t1);
t3 = derivative_q4_wrt_q2 ^ 2;
t4 = a4 * derivative_q4_wrt_q5 / 0.2e1;
t5 = -a5 * sin(q5) - t4 * t2;
t4 = a5 * cos(q5) + t4 * t1;
t6 = -m4 * a4 * derivative_q4_wrt_q2 * (-t4 * t1 + t2 * t5) / 0.2e1 + derivative_q4_wrt_q2 * Izz4 * derivative_q4_wrt_q5;
Mass_matrix_4 = [t3 * Izz4 + m4 * a4 ^ 2 * t3 * (t1 ^ 2 + t2 ^ 2) / 0.4e1 t6; t6 derivative_q4_wrt_q5 ^ 2 * Izz4 + (t4 ^ 2 + t5 ^ 2) * m4;];


% Summation index 5
Mass_matrix_5 = [0 0; 0 m5 * a5 ^ 2 /4 + Izz5 ];



Mass_matrix=Mass_matrix_2+Mass_matrix_3+Mass_matrix_4+Mass_matrix_5;







%%G Matrix




%--------------------------

t1 = a3 ^ 2;
t6 = derivative_q3_wrt_q2;
t9 = cos(q2);
t10 =q3;
t11 = cos(t10);
t13 = sin(q2);
t14 = sin(t10);
t19 = (t1 * m3 / 0.2e1 + (2 * Izz3)) * t6 + a2 * a3 * m3 * (t9 * t11 + t13 * t14);
t21 = derivative_q3_wrt_q2_q2;
t25 = derivative_q3_wrt_q2_q5;
t28 = derivative_q4_wrt_q2;
t30 = a4 ^ 2;
t33 = t30 * m4 + (4 * Izz4);
t34 = derivative_q4_wrt_q2_q2;
t39 = derivative_q4_wrt_q2_q5;
t50 = derivative_q3_wrt_q5;
G11= w2 * t19 * t21 / 0.2e1 + w5 * t19 * t25 / 0.2e1 + w2 * t28 * t33 * t34 / 0.4e1 + w5 * t28 * t33 * t39 / 0.4e1 - a2 * t6 * a3 * m3 * (-t13 * t11 + t9 * t14) * (w5 * t50 + w2 * t6 - w2) / 0.2e1;

%-------------------------------------------------------------------------

t1 = a3 ^ 2;
t6 = derivative_q3_wrt_q2;
t8 = a2 * a3;
t9 = cos(q2);
t10 = q3;
t11 = cos(t10);
t13 = sin(q2);
t14 = sin(t10);
t19 = (t1 * m3 / 0.2e1 + (2 * Izz3)) * t6 + t8 * m3 * (t9 * t11 + t13 * t14);
t21 = derivative_q3_wrt_q2_q5;
t25 = derivative_q3_wrt_q5_q5;
t28 = derivative_q4_wrt_q2;
t30 = a4 ^ 2;
t33 = t30 * m4 / 0.4e1 + Izz4;
t34 = derivative_q4_wrt_q2_q5;
t38 = derivative_q4_wrt_q5_q5;
t43 = derivative_q3_wrt_q5;
t47 = -t13 * t11 + t9 * t14;
t53 = q4;
t54 = sin(t53);
t55 = cos(q5);
t57 = cos(t53);
t58 = sin(q5);
t64 = t43 ^ 2;
G12 = w2 * t19 * t21 / 0.2e1 + w5 * t19 * t25 / 0.2e1 + w2 * t28 * t33 * t34 + w5 * t28 * t33 * t38 - a2 * w2 * a3 * t43 * m3 * t47 * t6 / 0.2e1 - (-a4 * a5 * m4 * (t54 * t55 - t57 * t58) * t28 + t8 * t64 * m3 * t47) * w5 / 0.2e1;


%---------------------------------------------------------------------------
t1 = a4 ^ 2;
t5 = derivative_q4_wrt_q5;
t8 = q4;
t9 = cos(t8);
t10 = cos(q5);
t12 = sin(t8);
t13 = sin(q5);
t19 = (t1 * m4 / 0.4e1 + Izz4) * t5 + a4 * a5 * m4 * (t9 * t10 + t12 * t13) / 0.2e1;
t21 = derivative_q4_wrt_q2_q2;
t24 = derivative_q4_wrt_q2_q5;
t26 = derivative_q3_wrt_q5;
t28 = a3 ^ 2;
t31 = t28 * m3 + 0.4e1 * Izz3;
t32 = derivative_q3_wrt_q2_q2;
t37 = derivative_q3_wrt_q2_q5;
t44 = cos(q2);
t45 = q3;
t46 = sin(t45);
t48 = sin(q2);
t49 = cos(t45);
t55 = derivative_q4_wrt_q2
G21 = w2 * t19 * t21 + w5 * t19 * t24 + w2 * t26 * t31 * t32 / 0.4e1 + w5 * t26 * t31 * t37 / 0.4e1 + a2 * w2 * a3 * t26 * m3 * (t44 * t46 - t48 * t49) / 0.2e1 - t55 * a4 * a5 * m4 * (t12 * t10 - t9 * t13) * (w5 * t5 + w2 * t55) / 0.2e1;

%--------------------------------------------------------------------------------------
t1 = a4 ^ 2;
t6 = derivative_q4_wrt_q5;
t9 = q4;
t10 = cos(t9);
t11 = cos(q5);
t13 = sin(t9);
t14 = sin(q5);
t19 = (t1 * m4 / 0.2e1 + (2 * Izz4)) * t6 + a4 * a5 * m4 * (t10 * t11 + t13 * t14);
t21 = derivative_q4_wrt_q2_q5;
t25 = derivative_q4_wrt_q5_q5;
t28 = derivative_q3_wrt_q5;
t30 = a3 ^ 2;
t33 = t30 * m3 + (4 * Izz3);
t34 = derivative_q3_wrt_q2_q5;
t39 = derivative_q3_wrt_q5_q5;
t49 = derivative_q4_wrt_q2;
G22 = w2 * t19 * t21 / 0.2e1 + w5 * t19 * t25 / 0.2e1 + w2 * t28 * t33 * t34 / 0.4e1 + w5 * t28 * t33 * t39 / 0.4e1 - a4 * t6 * a5 * m4 * (-t10 * t14 + t13 * t11) * (w2 * t49 + w5 * t6 - w5) / 0.2e1;



N=[G11,G12 ; G21,G22]*dq


%% Trajectory 


x=[0.5*a1+a5*cos(q5)+a4*cos(q4);
    a5*sin(q5)+a4*sin(q4)];  %2x1 Matrix


v=[-a5*sin(q5)*w5-a4*sin(q4)*w4 ; a5*cos(q5)*w5+a4*cos(q4)*w4];




%% Desired Position 
% 
% xd=[218+4*sin(t);250+4*cos(t)];
% vd=[4*cos(t);-4*sin(t)];
% ad=[-4*sin(t);-4*cos(t)];

% vd=diff(xd);
% ad=diff(vd);

% vd=[0;0];
% ad=[0;0];
%% Jacobian Matrix

%Matlab(J(1, 1), optimize);


t3 = sin(q2);
t5 = cos(q2);
t8 = sin(q5);
t12 = 2 * x(1,1);
t13 = a2 * t5;
t18 = cos(q5);
t19 = a5 * t18;
J11= 0.2e1 * ((x(1,1) + a1 / 0.2e1) * t3 - t5 * x(2,1)) * (a5 * t8 - x(2,1)) * a2 / (-(t12 - 0.2e1 * t13 + a1) * a5 * t8 + (t12 - 0.2e1 * t19 - a1) * a2 * t3 + 0.2e1 * x(2,1) * (-t13 + t19 + a1));






%Matlab(J(1, 2), optimize);
t3 = sin(q5);
t5 = cos(q5);
t9 = sin(q2);
t12 = 2 * x(1,1);
t13 = cos(q2);
t14 = a2 * t13;
t19 = a5 * t5;
J12= -0.2e1 * a5 * ((x(1,1) - a1 / 0.2e1) * t3 - t5 * x(2,1)) * (a2 * t9 - x(2,1)) / (-(t12 - 0.2e1 * t14 + a1) * a5 * t3 + (t12 - 0.2e1 * t19 - a1) * a2 * t9 + 0.2e1 * x(2,1) * (-t14 + t19 + a1));


%Matlab(J(2, 1), optimize);
t2 = cos(q5);
t3 = a5 * t2;
t6 = (4 * x(1,1)) - 0.4e1 * t3 - (2 * a1);
t8 = x(1,1) + a1 / 0.2e1;
t9 = sin(q2);
t11 = cos(q2);
t17 = sin(q5);
J21= t6 * (-t11 * x(2,1) + t8 * t9) * a2 / (t6 * a2 * t9 + 0.4e1 * a2 * (a5 * t17 - x(2,1)) * t11 + 0.4e1 * t3 * x(2,1) - 0.4e1 * a5 * t8 * t17 + 0.4e1 * a1 * x(2,1));

%Matlab(J(2, 2), optimize);

t1 = 4 * x(1,1);
t2 = cos(q2);
t3 = a2 * t2;
t5 = 2 * a1;
t7 = (t1 - 0.4e1 * t3 + t5) * a5;
t10 = sin(q5);
t12 = cos(q5);
t18 = sin(q2);
J22= -t7 * ((x(1,1) - a1 / 0.2e1) * t10 - t12 * x(2,1)) / (-t7 * t10 - 0.4e1 * t3 * x(2,1) - 0.4e1 * a5 * (a2 * t18 - x(2,1)) * t12 + (t1 - t5) * a2 * t18 + 0.4e1 * a1 * x(2,1));




J=[J11,J12 ; J21 ,J22];

detJ= det(J);






%% Derivative of Jacobian


t1 = v(1,1);
t2 = q2;
t3 = sin(t2);
t5 = x(1,1);
t6 = a1 / 0.2e1;
t7 = t5 + t6;
t8 = w2;
t10 = cos(t2);
t13 = x(2,1);
t15 = v(2,1);
t19 = q5;
t20 = sin(t19);
t22 = a5 * t20 - t13;
t23 = a2 * t10;
t25 = a5 * (t5 - t23 + t6);
t27 = cos(t19);
t28 = a5 * t27;
t30 = a2 * (t5 - t28 - t6);
t32 = -t23 + t28 + a1;
t34 = t13 * t32 - t25 * t20 + t30 * t3;
t35 = 0.1e1 / t34 / 0.2e1;
t41 = (-t10 * t13 + t7 * t3) * a2;
t42 = w5;
t43 = a5 * t42;
t52 = a2 * t8 * t3;
t58 = t43 * t20;
DJ11 = 0.2e1 * (t7 * t8 * t10 + t8 * t3 * t13 + t1 * t3 - t10 * t15) * a2 * t22 * t35 + 0.2e1 * t41 * (t43 * t27 - t15) * t35 - t41 * t22 / t34 ^ 2 * (-a5 * (t1 + t52) * t20 - t25 * t42 * t27 + a2 * (t1 + t58) * t3 + t30 * t8 * t10 + t15 * t32 + t13 * (t52 - t58));




t1 = v(1,1);
t2 = q5;
t3 = sin(t2);
t5 = x(1,1);
t6 = a1 / 0.2e1;
t7 = t5 - t6;
t8 = w5;
t10 = cos(t2);
t13 = x(2,1);
t15 = v(2,1);
t19 = q2;
t20 = sin(t19);
t22 = a2 * t20 - t13;
t23 = cos(t19);
t24 = a2 * t23;
t26 = a5 * (t5 - t24 + t6);
t28 = a5 * t10;
t30 = a2 * (t5 - t28 - t6);
t32 = -t24 + t28 + a1;
t34 = t13 * t32 + t30 * t20 - t26 * t3;
t35 = 0.1e1 / t34 / 0.2e1;
t41 = (-t10 * t13 + t7 * t3) * a5;
t42 = w2;
t43 = a2 * t42;
t51 = t43 * t20;
t58 = a5 * t8 * t3;
DJ12 = 0.2e1 * (t7 * t8 * t10 + t8 * t3 * t13 + t1 * t3 - t10 * t15) * a5 * t22 * t35 + 0.2e1 * t41 * (t43 * t23 - t15) * t35 - t41 * t22 / t34 ^ 2 * (-a5 * (t1 + t51) * t3 - t26 * t8 * t10 + a2 * (t1 + t58) * t20 + t30 * t42 * t23 + t15 * t32 + t13 * (t51 - t58));




t1 = v(1,1);
t2 = q2;
t3 = sin(t2);
t5 = x(1,1);
t6 = a1 / 0.2e1;
t7 = t5 + t6;
t8 = w2;
t10 = cos(t2);
t12 = t8 * t3;
t13 = x(2,1);
t15 = v(2,1);
t19 = q5;
t20 = cos(t19);
t21 = a5 * t20;
t22 = t5 - t21 - t6;
t23 = a2 * t22;
t25 = sin(t19);
t28 = a2 * (a5 * t25 - t13);
t31 = t7 * a5;
t34 = a1 * t13 + t28 * t10 + t21 * t13 + t23 * t3 - t31 * t25;
t35 = 0.1e1 / t34 / 0.4e1;
t41 = (-t10 * t13 + t7 * t3) * a2;
t42 = w5;
t43 = a5 * t42;
t45 = t43 * t25 + t1;
DJ21 = 0.4e1 * (t7 * t8 * t10 + t1 * t3 - t10 * t15 + t12 * t13) * a2 * t22 * t35 + 0.4e1 * t41 * t45 * t35 - t41 * t22 / t34 ^ 2 * (a2 * t45 * t3 + t23 * t8 * t10 + a2 * (t43 * t20 - t15) * t10 - t28 * t12 - t42 * t25 * a5 * t13 + t21 * t15 - t1 * a5 * t25 - t31 * t42 * t20 + a1 * t15);



t1 = v(1,1);
t2 = q5;
t3 = sin(t2);
t5 = x(1,1);
t6 = a1 / 0.2e1;
t7 = t5 - t6;
t8 = w5;
t10 = cos(t2);
t12 = t8 * t3;
t13 = x(2,1);
t15 = v(2,1);
t19 = q2;
t20 = cos(t19);
t21 = a2 * t20;
t22 = t5 - t21 + t6;
t23 = a5 * t22;
t26 = sin(t19);
t29 = a5 * (a2 * t26 - t13);
t31 = a2 * t7;
t34 = a1 * t13 - t29 * t10 - t21 * t13 - t23 * t3 + t31 * t26;
t35 = 0.1e1 / t34 / 0.4e1;
t41 = (-t10 * t13 + t7 * t3) * a5;
t42 = w2;
t43 = a2 * t42;
t45 = t43 * t26 + t1;
DJ22 = -0.4e1 * (t7 * t8 * t10 + t1 * t3 - t10 * t15 + t12 * t13) * a5 * t22 * t35 - 0.4e1 * t41 * t45 * t35 + t41 * t22 / t34 ^ 2 * (-a5 * t45 * t3 - t23 * t8 * t10 + t42 * t26 * a2 * t13 - t21 * t15 - a5 * (t43 * t20 - t15) * t10 + t29 * t12 + a2 * t1 * t26 + t31 * t42 * t20 + a1 * t15);


dJ=[DJ11 ,DJ12 ; DJ21 , DJ22];

%% 

invJ=inv(J);
e=x-xd;     % 2x2 Matrix


Torque=Mass_matrix*(invJ*(ad+Kv*(vd-v)+Kp*(xd-x)-dJ*dq))+N;


% u=invJ*(diff(xd)-K*e);    % 2x1 Matrix
